simulink model "Hydraulic_Actuator"  (R2021a)
settings: Solver=ode4  StartTime=0.0  StopTime=0.5  FixedStep=0.0005  RelTol=1e-3
values from neighbouring files (symbols this model uses):
  Ap = 20.44*10^(-4)    (= 0.002044)    [parameter.m]
  beta = 9.81*10^(8)    (= 981000000)    [parameter.m]
  F = 2.044*10^(3)    (= 2044)    [parameter.m]
  M = 1000    [parameter.m]
  P1i = Po    (= 10000000)    [parameter.m]
  P2i = Po    (= 10000000)    [parameter.m]
  Vo = 1.063*10^(-4)    (= 0.0001063)    [parameter.m]
settings Model: Creator=nehab  LastModifiedBy=nehab

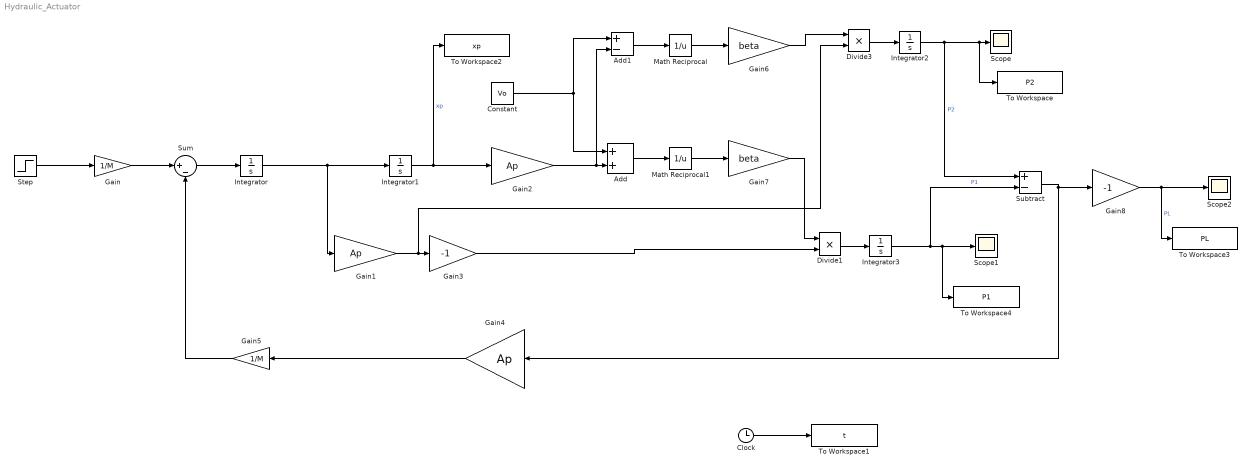
== system Hydraulic_Actuator ==
  Add : Sum
  Add1 : Sum  Inputs=+-
  Clock : Clock
  Constant : Constant  Value=Vo
  Divide1 : Product  Inputs=**
  Divide3 : Product  Inputs=**
  Gain : Gain  Gain=1/M
  Gain1 : Gain  Gain=Ap
  Gain2 : Gain  Gain=Ap
  Gain3 : Gain  Gain=-1
  Gain4 : Gain  Gain=Ap
  Gain5 : Gain  Gain=1/M
  Gain6 : Gain  Gain=beta
  Gain7 : Gain  Gain=beta
  Gain8 : Gain  Gain=-1
  Integrator : Integrator
  Integrator1 : Integrator
  Integrator2 : Integrator  InitialCondition=P2i
  Integrator3 : Integrator  InitialCondition=P1i
  Math Reciprocal : Math  Operator=reciprocal  SignedPower=on  SaturateOnIntegerOverflow=on
  Math Reciprocal1 : Math  Operator=reciprocal  SignedPower=on  SaturateOnIntegerOverflow=on
  Scope : Scope
  Scope1 : Scope
  Scope2 : Scope
  Step : Step  Time=0  After=F  SampleTime=0
  Subtract : Sum  Inputs=+-
  Sum : Sum  Inputs=|+-
  To Workspace : ToWorkspace  VariableName=P2  SampleTime=-1
  To Workspace1 : ToWorkspace  VariableName=t  SampleTime=-1
  To Workspace2 : ToWorkspace  VariableName=xp  SampleTime=-1
  To Workspace3 : ToWorkspace  VariableName=PL  SampleTime=-1
  To Workspace4 : ToWorkspace  VariableName=P1  SampleTime=-1
  wires:
  Step/1 -> Gain/1
  Gain/1 -> Sum/1
  Sum/1 -> Integrator/1
  Integrator/1 -> Gain1/1, Integrator1/1
  Integrator1/1 -> To Workspace2/1, Gain2/1  "xp"
  Gain2/1 -> Add1/2, Add/2
  Constant/1 -> Add1/1, Add/1
  Gain1/1 -> Divide3/2, Gain3/1
  Gain3/1 -> Divide1/2
  Add1/1 -> Math Reciprocal/1
  Divide3/1 -> Integrator2/1
  Divide1/1 -> Integrator3/1
  Subtract/1 -> Gain8/1, Gain4/1
  Gain4/1 -> Gain5/1
  Gain5/1 -> Sum/2
  Add/1 -> Math Reciprocal1/1
  Math Reciprocal/1 -> Gain6/1
  Math Reciprocal1/1 -> Gain7/1
  Gain6/1 -> Divide3/1
  Gain7/1 -> Divide1/1
  Integrator2/1 -> To Workspace/1, Scope/1, Subtract/1  "P2"
  Integrator3/1 -> To Workspace4/1, Scope1/1, Subtract/2  "P1"
  Gain8/1 -> To Workspace3/1, Scope2/1  "PL"
  Clock/1 -> To Workspace1/1
